simulink model "RS_7"  (R2018a)
settings: Solver=VariableStepAuto  StartTime=0.0  StopTime=10.0  RelTol=1e-3
values from neighbouring files (symbols this model uses):
  BER = ber(ii)    [CRC_88.m]    (also in RS_77.m)
undefined symbols (not defined in the file or in its folder): rsgenpoly
libraries: commblkcod2 x2, commchan3 x1, commsink2 x1, commrandsrc3 x1
settings Model: Creator=sdf  LastModifiedBy=sdf

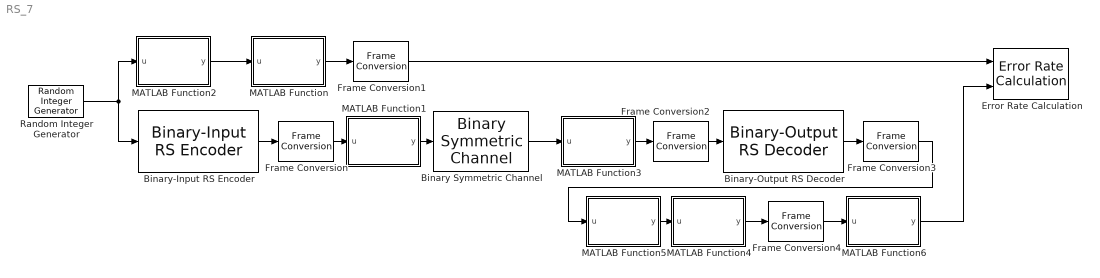
== system RS_7 ==
  Binary Symmetric Channel : commchan3/Binary Symmetric Channel  P=BER  s=71  E=off  outDtype=double
      settings: SourceProductName=Communications System Toolbox  SourceProductBaseCode=CM
  Binary-Input RS Encoder : commblkcod2/Binary-Input RS Encoder  n=15  k=11  specShortening=off  shortenedK=3  specGenPoly=off  genPoly=rsgenpoly(7, 3, [], [], 'double')  specPrimPoly=off  prPoly='X^3 + X + 1'  specPuncture=off  punctVec=[ones(2,1); zeros(2,1)]  outDType=Same as input
      settings: SourceProductName=Communications System Toolbox  SourceProductBaseCode=CM
  Binary-Output RS Decoder : commblkcod2/Binary-Output RS Decoder  n=15  k=11  specShortening=off  shortenedK=3  specGenPoly=off  genPoly=rsgenpoly(7, 3, [], [], 'double')  specPrimPoly=off  prPoly='X^3 + X + 1'  specPuncture=off  punctVec=[ones(2,1); zeros(2,1)]  specErasurePort=off  showNumErr=off  outDType=Same as input
      settings: SourceProductName=Communications System Toolbox  SourceProductBaseCode=CM
  Error Rate Calculation : commsink2/Error Rate Calculation  N=0  st_delay=0  cp_mode=Entire frame  subframe=[]  PMode=Workspace  WsName=BER  RsMode2=off  stop=off  numErr=100  maxBits=1e6
  Frame Conversion : FrameConversion  OutFrame=Sample-based
  Frame Conversion1 : FrameConversion  OutFrame=Sample-based
  Frame Conversion2 : FrameConversion
  Frame Conversion3 : FrameConversion  OutFrame=Sample-based
  Frame Conversion4 : FrameConversion
  MATLAB Function : MATLAB Function  TreatAsAtomicUnit=on
  MATLAB Function1 : MATLAB Function  TreatAsAtomicUnit=on
  MATLAB Function2 : MATLAB Function  TreatAsAtomicUnit=on
  MATLAB Function3 : MATLAB Function  TreatAsAtomicUnit=on
  MATLAB Function4 : MATLAB Function  TreatAsAtomicUnit=on
  MATLAB Function5 : MATLAB Function  TreatAsAtomicUnit=on
  MATLAB Function6 : MATLAB Function  TreatAsAtomicUnit=on
  Random Integer Generator : commrandsrc3/Random Integer Generator  SetSize=16  SeedSource=Parameter  Seed=37  SampleTime=1/110000  SamplesPerFrame=11  OutputDataType=double  SimulateUsing=Interpreted execution
  wires:
  Binary-Input RS Encoder/1 -> Frame Conversion/1
  Frame Conversion/1 -> MATLAB Function1/1(u)
  MATLAB Function2/1(y) -> MATLAB Function/1(u)
  MATLAB Function/1(y) -> Frame Conversion1/1
  MATLAB Function1/1(y) -> Binary Symmetric Channel/1
  MATLAB Function3/1(y) -> Frame Conversion2/1
  Frame Conversion2/1 -> Binary-Output RS Decoder/1
  Binary-Output RS Decoder/1 -> Frame Conversion3/1
  Frame Conversion3/1 -> MATLAB Function5/1(u)
  MATLAB Function5/1(y) -> MATLAB Function4/1(u)
  MATLAB Function4/1(y) -> Frame Conversion4/1
  Frame Conversion4/1 -> MATLAB Function6/1(u)
  Binary Symmetric Channel/1 -> MATLAB Function3/1(u)
  Frame Conversion1/1 -> Error Rate Calculation/1
  MATLAB Function6/1(y) -> Error Rate Calculation/2
  Random Integer Generator/1 -> Binary-Input RS Encoder/1, MATLAB Function2/1(u)

== matlab function RS_7/MATLAB Function1 ==
  data: u input; y output
function y = fcn(u)

y = de2bi(u,4,'left-msb');

== matlab function RS_7/MATLAB Function ==
  data: u input; y output
function y = fcn(u)

y = reshape(u.',44,1);

== matlab function RS_7/MATLAB Function2 ==
  data: u input; y output
function y = fcn(u)

y = de2bi(u,4,'left-msb');

== matlab function RS_7/MATLAB Function3 ==
  data: u input; y output
function y = fcn(u)

y = bi2de(u,'left-msb');

== matlab function RS_7/MATLAB Function4 ==
  data: u input; y output
function y = fcn(u)

y = reshape(u.',44,1);

== matlab function RS_7/MATLAB Function5 ==
  data: u input; y output
function y = fcn(u)

y = de2bi(u,4,'left-msb');

== matlab function RS_7/MATLAB Function6 ==
  data: u input; y output
function y = fcn(u)

y = reshape(u.',44,1);
